simulink model "Slew_Manuever"  (R2021b)
settings: Solver=VariableStepAuto  StartTime=0.0  StopTime=10.0  RelTol=1e-3
undefined symbols (not defined in the file or in its folder): k1, k2
libraries: matrix_library x1
settings Model: Creator=hp  LastModifiedBy=hp

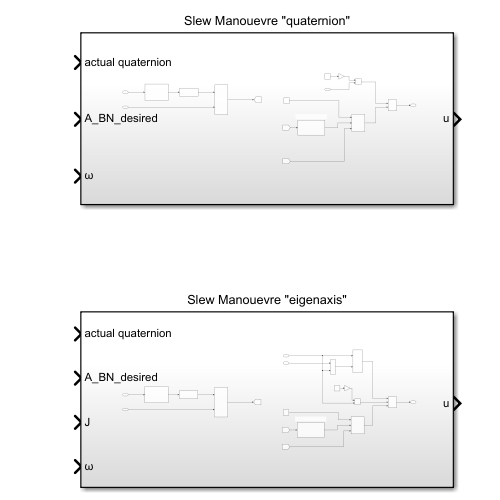
[thumbnail: Simulink's stored preview of the top-level diagram]
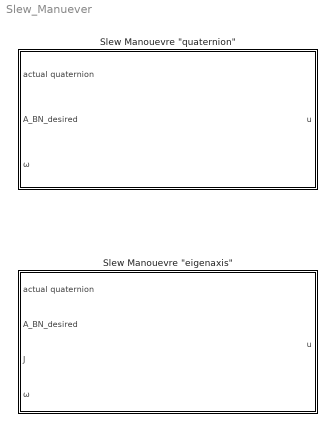
== system Slew_Manuever ==
  "Slew Manouevre \"eigenaxis\"" : Subsystem
  "Slew Manouevre \"quaternion\"" : Subsystem

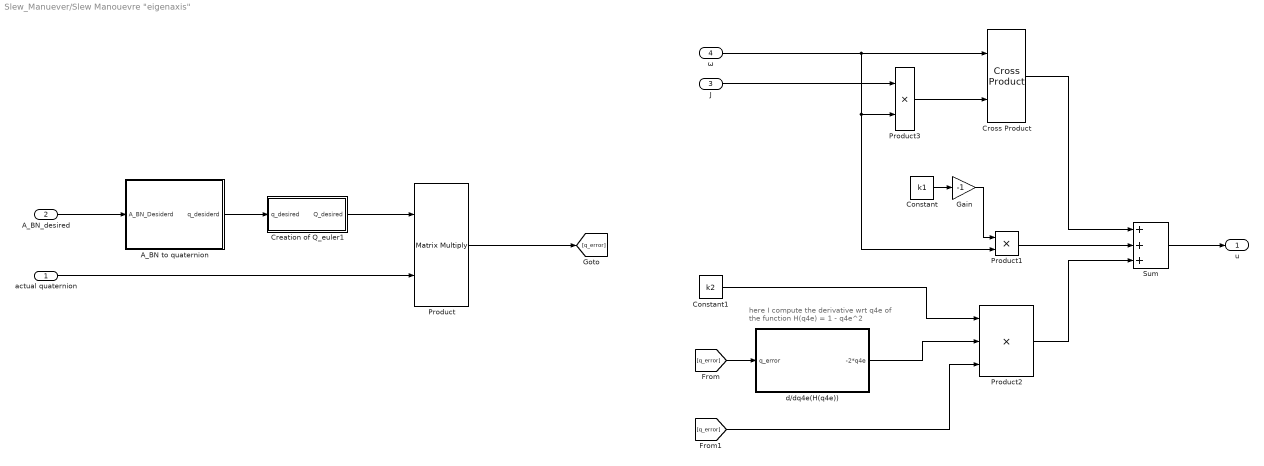
== system Slew_Manuever/Slew Manouevre "eigenaxis" ==
  note: here I compute the derivative wrt q4e
      | of the function H(q4e) = 1 - q4e^2
  actual quaternion : Inport
  A_BN_desired : Inport  Port=2
  J : Inport  Port=3
  ω : Inport  Port=4
  A_BN to quaternion : Subsystem
  Constant : Constant  Value=k1
  Constant1 : Constant  Value=k2
  Creation of Q_euler1 : Subsystem
  Cross Product : matrix_library/Cross Product
      settings: SourceProductBaseCode=SL
  Gain : Gain  Gain=-1
  Product : Product  Multiplication=Matrix(*)
  Product1 : Product
  Product2 : Product  Inputs=3
  Product3 : Product
  Sum : Sum  Inputs=|+|+|+|
  d/dq4e(H(q4e)) : Subsystem
  u : Outport
  wires:
  Sum/1 -> u/1
  Product2/1 -> Sum/3
  Product1/1 -> Sum/2
  [q_error] -> Product2/3
  d/dq4e(H(q4e))/1(-2*q4e) -> Product2/2
  Constant1/1 -> Product2/1
  ω/1 -> Product1/2, Product3/2, Cross Product/1
  Gain/1 -> Product1/1
  Constant/1 -> Gain/1
  [q_error] -> d/dq4e(H(q4e))/1(q_error)
  A_BN to quaternion/1(q_desiderd) -> Creation of Q_euler1/1(q_desired)
  A_BN_desired/1 -> A_BN to quaternion/1(" A_BN_Desiderd")
  Product/1 -> [q_error]
  Creation of Q_euler1/1(Q_desired) -> Product/1
  actual quaternion/1 -> Product/2
  J/1 -> Product3/1
  Product3/1 -> Cross Product/2
  Cross Product/1 -> Sum/1

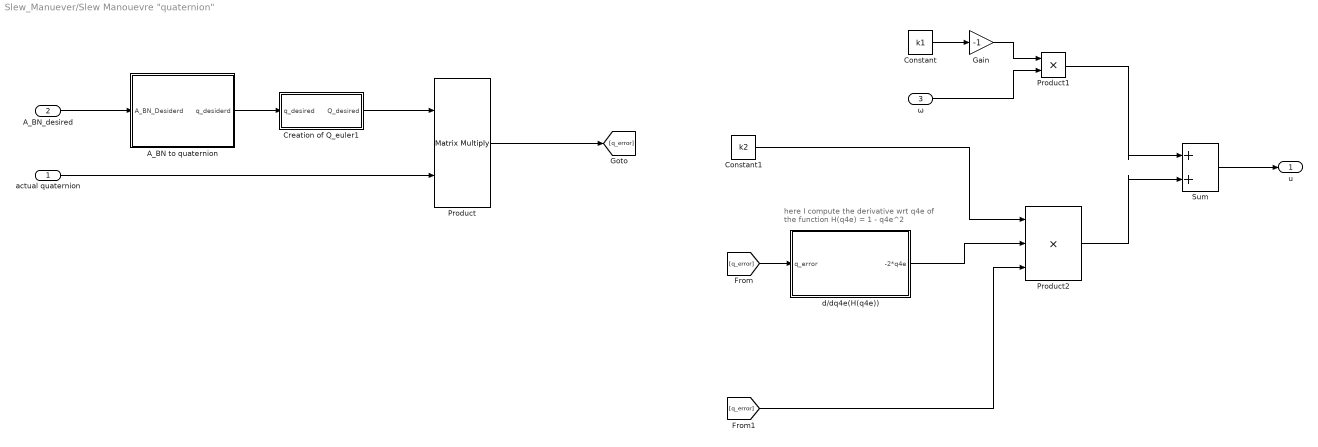
== system Slew_Manuever/Slew Manouevre "quaternion" ==
  note: here I compute the derivative wrt q4e
      | of the function H(q4e) = 1 - q4e^2
  actual quaternion : Inport
  A_BN_desired : Inport  Port=2
  ω : Inport  Port=3
  A_BN to quaternion : Subsystem
  Constant : Constant  Value=k1
  Constant1 : Constant  Value=k2
  Creation of Q_euler1 : Subsystem
  Gain : Gain  Gain=-1
  Product : Product  Multiplication=Matrix(*)
  Product1 : Product
  Product2 : Product  Inputs=3
  Sum : Sum  Inputs=|+|+|
  d/dq4e(H(q4e)) : Subsystem
  u : Outport
  wires:
  actual quaternion/1 -> Product/2
  Creation of Q_euler1/1(Q_desired) -> Product/1
  Product/1 -> [q_error]
  A_BN_desired/1 -> A_BN to quaternion/1(" A_BN_Desiderd")
  A_BN to quaternion/1(q_desiderd) -> Creation of Q_euler1/1(q_desired)
  [q_error] -> d/dq4e(H(q4e))/1(q_error)
  Constant/1 -> Gain/1
  Gain/1 -> Product1/1
  ω/1 -> Product1/2
  Constant1/1 -> Product2/1
  d/dq4e(H(q4e))/1(-2*q4e) -> Product2/2
  [q_error] -> Product2/3
  Product1/1 -> Sum/1
  Product2/1 -> Sum/2
  Sum/1 -> u/1

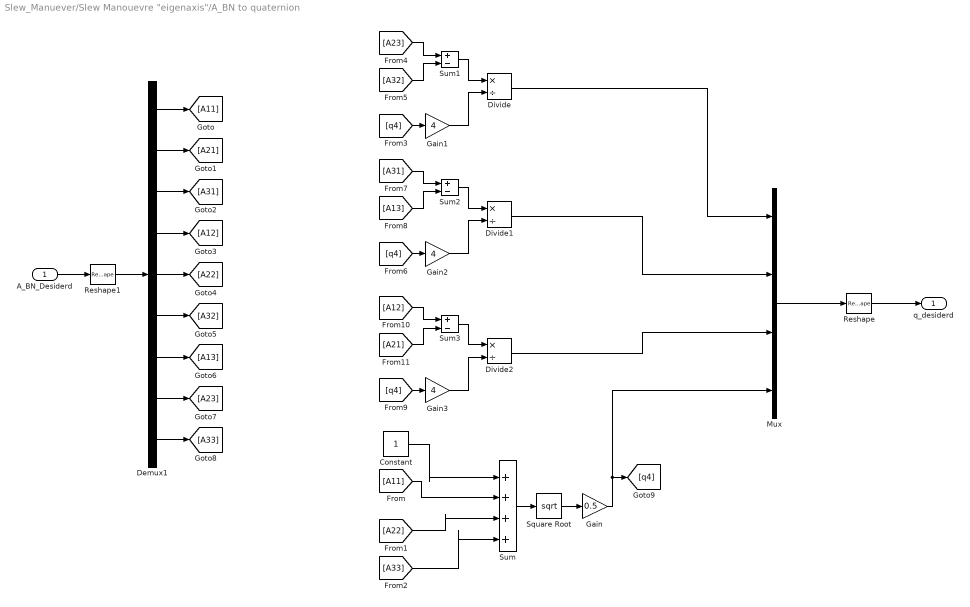
== system Slew_Manuever/Slew Manouevre "eigenaxis"/A_BN to quaternion ==
  " A_BN_Desiderd" : Inport
  Constant : Constant
  Demux1 : Demux  Outputs=9
  Divide : Product  Inputs=*/
  Divide1 : Product  Inputs=*/
  Divide2 : Product  Inputs=*/
  Gain : Gain  Gain=0.5
  Gain1 : Gain  Gain=4
  Gain2 : Gain  Gain=4
  Gain3 : Gain  Gain=4
  Mux : Mux
  Reshape : Reshape  OutputDimensionality=Column vector (2-D)
  Reshape1 : Reshape  OutputDimensionality=Column vector (2-D)
  Square Root : Sqrt  SaturateOnIntegerOverflow=on
  Sum : Sum  Inputs=|+|+|+|+|
  Sum1 : Sum  Inputs=|+|-|
  Sum2 : Sum  Inputs=|+|-|
  Sum3 : Sum  Inputs=|+|-|
  q_desiderd : Outport
  wires:
  Demux1/7 -> [A13]
  Demux1/3 -> [A31]
  Demux1/9 -> [A33]
  Demux1/5 -> [A22]
  Demux1/8 -> [A23]
  [A21] -> Sum3/2
  Reshape1/1 -> Demux1/1
  [A11] -> Sum/2
  Demux1/1 -> [A11]
  " A_BN_Desiderd"/1 -> Reshape1/1
  [A23] -> Sum1/1
  [A22] -> Sum/3
  Demux1/6 -> [A32]
  Demux1/2 -> [A21]
  [A32] -> Sum1/2
  Sum/1 -> Square Root/1
  Constant/1 -> Sum/1
  Square Root/1 -> Gain/1
  [q4] -> Gain1/1
  Divide1/1 -> Mux/2
  Sum1/1 -> Divide/1
  [A31] -> Sum2/1
  Sum2/1 -> Divide1/1
  Gain2/1 -> Divide1/2
  Sum3/1 -> Divide2/1
  Divide2/1 -> Mux/3
  [A12] -> Sum3/1
  Demux1/4 -> [A12]
  Gain/1 -> [q4], Mux/4
  Reshape/1 -> q_desiderd/1
  Gain3/1 -> Divide2/2
  [A13] -> Sum2/2
  [q4] -> Gain2/1
  Divide/1 -> Mux/1
  Gain1/1 -> Divide/2
  [q4] -> Gain3/1
  Mux/1 -> Reshape/1
  [A33] -> Sum/4

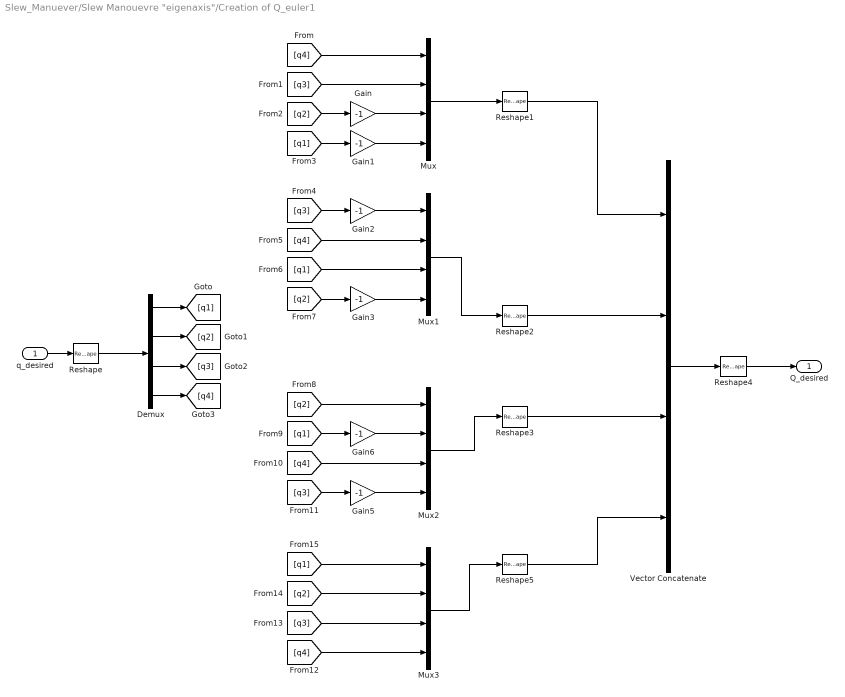
== system Slew_Manuever/Slew Manouevre "eigenaxis"/Creation of Q_euler1 ==
  q_desired : Inport
  Demux : Demux
  Gain{,1..3,5..6} (6 alike) : Gain  Gain=-1
  Mux{,1..3} (4 alike) : Mux
  Reshape : Reshape  OutputDimensionality=Column vector (2-D)
  Reshape{1..3,5} (4 alike) : Reshape  OutputDimensionality=Row vector (2-D)
  Reshape4 : Reshape  OutputDimensionality=Customize  OutputDimensions=[4,4]
  Vector Concatenate : Concatenate  NumInputs=4
  Q_desired : Outport
  wires:
  [q3] -> Mux3/3
  [q4] -> Mux3/4
  [q2] -> Mux3/2
  Mux3/1 -> Reshape5/1
  [q1] -> Mux3/1
  Reshape5/1 -> Vector Concatenate/4
  q_desired/1 -> Reshape/1
  Reshape/1 -> Demux/1
  Demux/1 -> [q1]
  Demux/2 -> [q2]
  Demux/3 -> [q3]
  Demux/4 -> [q4]
  [q2] -> Gain/1
  [q1] -> Gain1/1
  Gain1/1 -> Mux/4
  [q4] -> Mux/1
  [q3] -> Mux/2
  Gain/1 -> Mux/3
  Mux/1 -> Reshape1/1
  [q1] -> Mux1/3
  [q2] -> Gain3/1
  Mux1/1 -> Reshape2/1
  Gain3/1 -> Mux1/4
  [q4] -> Mux2/3
  [q2] -> Mux2/1
  [q3] -> Gain5/1
  Mux2/1 -> Reshape3/1
  Gain5/1 -> Mux2/4
  [q3] -> Gain2/1
  Gain2/1 -> Mux1/1
  [q4] -> Mux1/2
  [q1] -> Gain6/1
  Gain6/1 -> Mux2/2
  Reshape1/1 -> Vector Concatenate/1
  Reshape2/1 -> Vector Concatenate/2
  Reshape3/1 -> Vector Concatenate/3
  Vector Concatenate/1 -> Reshape4/1
  Reshape4/1 -> Q_desired/1

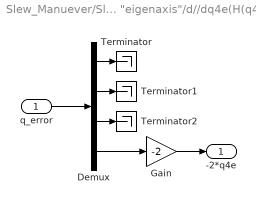
== system Slew_Manuever/Slew Manouevre "eigenaxis"/d//dq4e(H(q4e)) ==
  q_error : Inport
  Demux : Demux
  Gain : Gain  Gain=-2
  Terminator : Terminator
  Terminator1 : Terminator
  Terminator2 : Terminator
  -2*q4e : Outport
  wires:
  Gain/1 -> -2*q4e/1
  q_error/1 -> Demux/1
  Demux/4 -> Gain/1
  Demux/1 -> Terminator/1
  Demux/3 -> Terminator2/1
  Demux/2 -> Terminator1/1

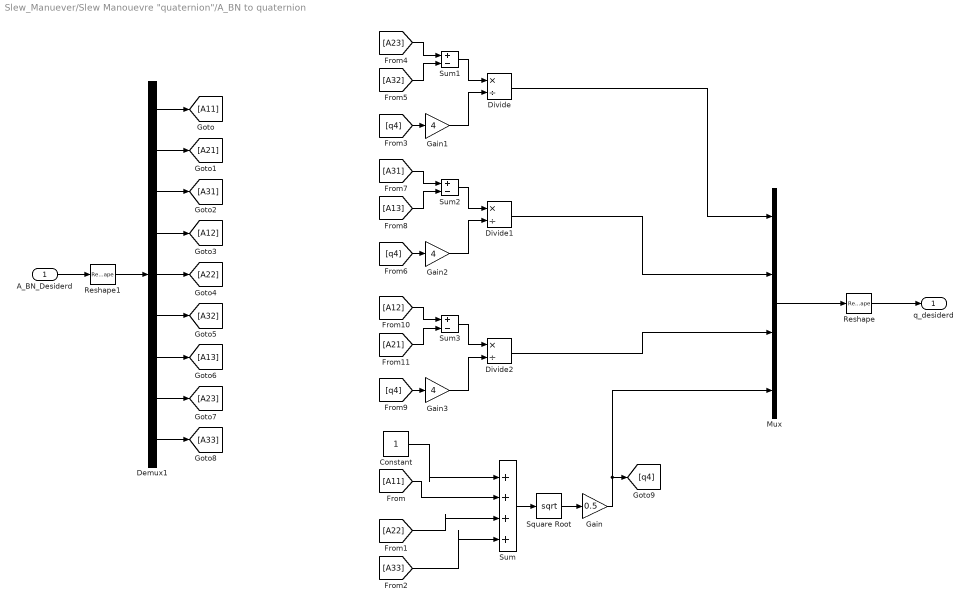
== system Slew_Manuever/Slew Manouevre "quaternion"/A_BN to quaternion ==
  " A_BN_Desiderd" : Inport
  Constant : Constant
  Demux1 : Demux  Outputs=9
  Divide : Product  Inputs=*/
  Divide1 : Product  Inputs=*/
  Divide2 : Product  Inputs=*/
  Gain : Gain  Gain=0.5
  Gain1 : Gain  Gain=4
  Gain2 : Gain  Gain=4
  Gain3 : Gain  Gain=4
  Mux : Mux
  Reshape : Reshape  OutputDimensionality=Column vector (2-D)
  Reshape1 : Reshape  OutputDimensionality=Column vector (2-D)
  Square Root : Sqrt  SaturateOnIntegerOverflow=on
  Sum : Sum  Inputs=|+|+|+|+|
  Sum1 : Sum  Inputs=|+|-|
  Sum2 : Sum  Inputs=|+|-|
  Sum3 : Sum  Inputs=|+|-|
  q_desiderd : Outport
  wires:
  [A33] -> Sum/4
  Mux/1 -> Reshape/1
  [q4] -> Gain3/1
  Gain1/1 -> Divide/2
  Divide/1 -> Mux/1
  [q4] -> Gain2/1
  [A13] -> Sum2/2
  Gain3/1 -> Divide2/2
  Reshape/1 -> q_desiderd/1
  Gain/1 -> Mux/4, [q4]
  Demux1/4 -> [A12]
  [A12] -> Sum3/1
  Divide2/1 -> Mux/3
  Sum3/1 -> Divide2/1
  Gain2/1 -> Divide1/2
  Sum2/1 -> Divide1/1
  [A31] -> Sum2/1
  Sum1/1 -> Divide/1
  Divide1/1 -> Mux/2
  [q4] -> Gain1/1
  Square Root/1 -> Gain/1
  Constant/1 -> Sum/1
  Sum/1 -> Square Root/1
  [A32] -> Sum1/2
  Demux1/2 -> [A21]
  Demux1/6 -> [A32]
  [A22] -> Sum/3
  [A23] -> Sum1/1
  " A_BN_Desiderd"/1 -> Reshape1/1
  Demux1/1 -> [A11]
  [A11] -> Sum/2
  Reshape1/1 -> Demux1/1
  [A21] -> Sum3/2
  Demux1/8 -> [A23]
  Demux1/5 -> [A22]
  Demux1/9 -> [A33]
  Demux1/3 -> [A31]
  Demux1/7 -> [A13]

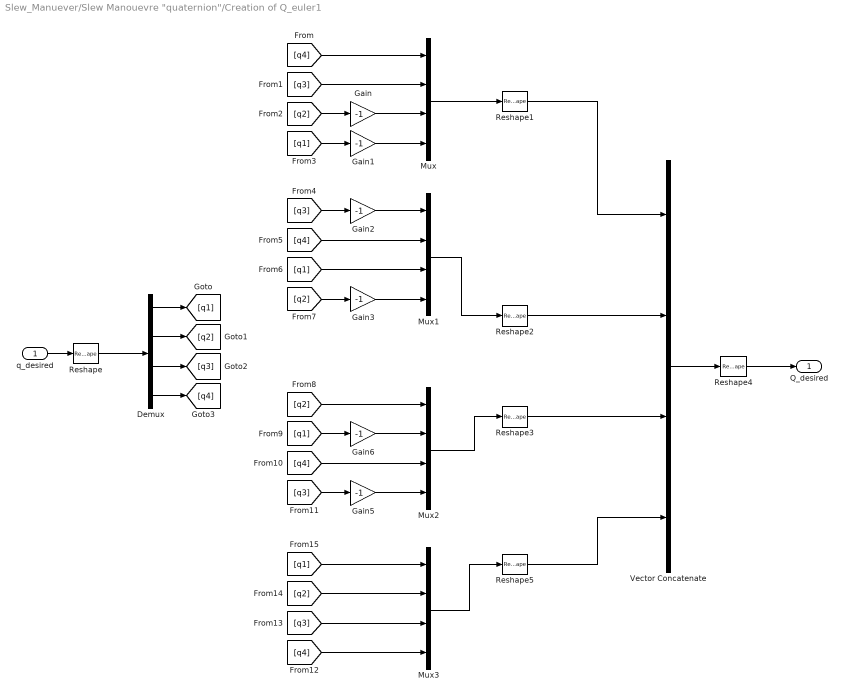
== system Slew_Manuever/Slew Manouevre "quaternion"/Creation of Q_euler1 ==
  q_desired : Inport
  Demux : Demux
  Gain{,1..3,5..6} (6 alike) : Gain  Gain=-1
  Mux{,1..3} (4 alike) : Mux
  Reshape : Reshape  OutputDimensionality=Column vector (2-D)
  Reshape{1..3,5} (4 alike) : Reshape  OutputDimensionality=Row vector (2-D)
  Reshape4 : Reshape  OutputDimensionality=Customize  OutputDimensions=[4,4]
  Vector Concatenate : Concatenate  NumInputs=4
  Q_desired : Outport
  wires:
  Reshape4/1 -> Q_desired/1
  Vector Concatenate/1 -> Reshape4/1
  Reshape3/1 -> Vector Concatenate/3
  Reshape2/1 -> Vector Concatenate/2
  Reshape1/1 -> Vector Concatenate/1
  Gain6/1 -> Mux2/2
  [q1] -> Gain6/1
  [q4] -> Mux1/2
  Gain2/1 -> Mux1/1
  [q3] -> Gain2/1
  Gain5/1 -> Mux2/4
  Mux2/1 -> Reshape3/1
  [q3] -> Gain5/1
  [q2] -> Mux2/1
  [q4] -> Mux2/3
  Gain3/1 -> Mux1/4
  Mux1/1 -> Reshape2/1
  [q2] -> Gain3/1
  [q1] -> Mux1/3
  Mux/1 -> Reshape1/1
  Gain/1 -> Mux/3
  [q3] -> Mux/2
  [q4] -> Mux/1
  Gain1/1 -> Mux/4
  [q1] -> Gain1/1
  [q2] -> Gain/1
  Demux/4 -> [q4]
  Demux/3 -> [q3]
  Demux/2 -> [q2]
  Demux/1 -> [q1]
  Reshape/1 -> Demux/1
  q_desired/1 -> Reshape/1
  Reshape5/1 -> Vector Concatenate/4
  [q1] -> Mux3/1
  Mux3/1 -> Reshape5/1
  [q2] -> Mux3/2
  [q4] -> Mux3/4
  [q3] -> Mux3/3

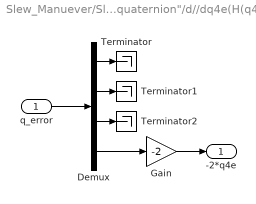
== system Slew_Manuever/Slew Manouevre "quaternion"/d//dq4e(H(q4e)) ==
  q_error : Inport
  Demux : Demux
  Gain : Gain  Gain=-2
  Terminator : Terminator
  Terminator1 : Terminator
  Terminator2 : Terminator
  -2*q4e : Outport
  wires:
  Demux/2 -> Terminator1/1
  Demux/3 -> Terminator2/1
  Demux/1 -> Terminator/1
  Demux/4 -> Gain/1
  q_error/1 -> Demux/1
  Gain/1 -> -2*q4e/1
